simulink model "pid_control_aerobot"  (R2024a)
settings: Solver=ode1  StartTime=0.0  StopTime=inf  FixedStep=0.01  RelTol=1e-3
undefined symbols (not defined in the file or in its folder): DiscIntNeverNeededParam, pin_number, state
libraries: ros2lib x14, simulink x2, sharedtransform x1
settings Model: SimulationMode=external  Creator=dsai9  LastModifiedBy=dsai9
settings OptimizationCC: EnhancedBackFolding=on  PassReuseOutputArgsAs=Individual arguments  ZeroExternalMemoryAtStartup=off  ZeroInternalMemoryAtStartup=off  MaxStackSize=64  OptimizeBlockOrder=speed  DifferentSizesBufferReuse=on  OptimizationCustomize=off  EfficientTunableParamExpr=on
settings DebuggingCC: ParameterTunabilityLossMsg=error
settings HardwareCC: ProdBitPerLong=64  ProdLargestAtomicInteger=LongLong  ProdLargestAtomicFloat=Double  ProdLongLongMode=on  ProdHWDeviceType=ARM Compatible->ARM Cortex-A (64-bit)
settings SFSimCC: MATLABDynamicMemAlloc=off
settings RTWCC: Description=Embedded Coder  SystemTargetFile=ert.tlc  HardwareBoard=Robot Operating System 2 (ROS 2)  TLCOptions="-aInlineSetEventsForThisBaseRateFcn=TLC_FALSE -aSuppressMultiTaskScheduler=TLC_FALSE  -aRateBasedStepFcn=0"  TemplateMakefile=ert_default_tmf  Toolchain=Colcon Tools  TargetLang=C++  GPUComputeCapability=3.5
settings CodeAppCC: ForceParamTrailComments=on  IgnoreCustomStorageClasses=off  OperatorAnnotations=on  SimulinkDataObjDesc=on  SFDataObjDesc=on  InsertBlockDesc=on
settings ERTTargetCC: TargetLangStandard=C++11 (ISO)  ExtMode=on  ExtModeMexArgs='192.168.0.122' 0 17725  RootIOFormat=Structure reference

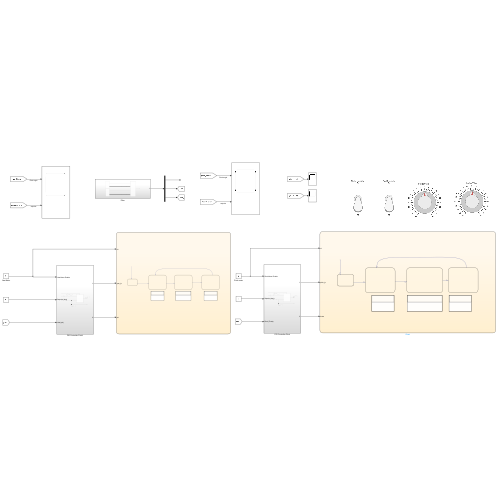
[thumbnail: Simulink's stored preview of the top-level diagram]
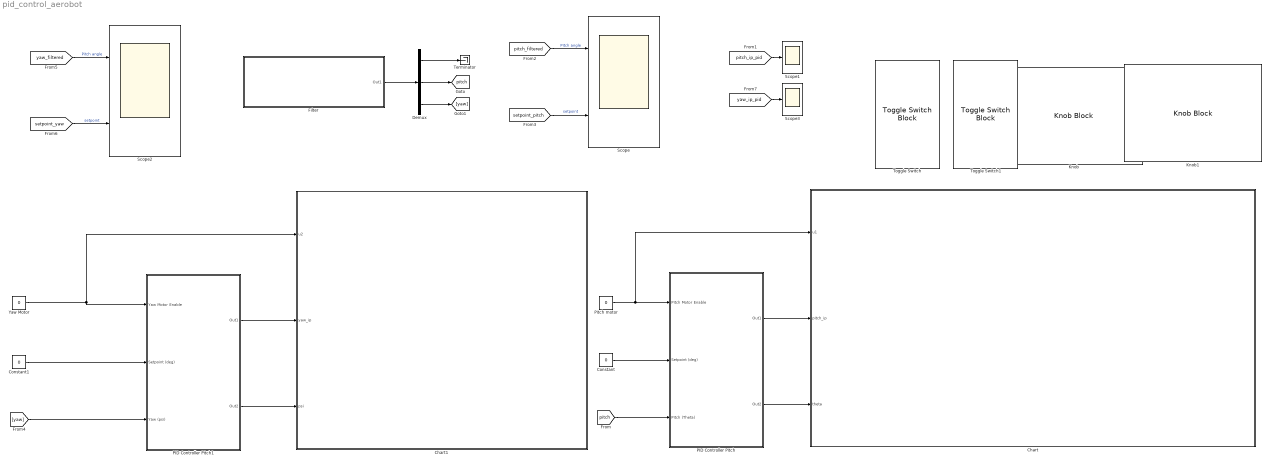
== system pid_control_aerobot ==
  Chart : Stateflow chart  TreatAsAtomicUnit=on
  Chart1 : Stateflow chart  TreatAsAtomicUnit=on
  Constant : Constant  Value=0
  Constant1 : Constant  Value=0
  Demux : Demux  Outputs=3
  Filter : Subsystem
  Knob : KnobBlock  ScaleMin=-40  ScaleMax=40
  Knob1 : KnobBlock  ScaleMin=-40  ScaleMax=40
  PID Controller Pitch : Subsystem
  PID Controller Pitch1 : Subsystem
  Pitch motor : Constant  Value=0  OutDataTypeStr=boolean
  Scope : Scope  NumInputPorts=2
  Scope1 : Scope
  Scope2 : Scope  NumInputPorts=2
  Scope3 : Scope
  Terminator : Terminator
  Toggle Switch : ToggleSwitchBlock
      settings: Values={{'Off', 'On'}, [0 1]}
  Toggle Switch1 : ToggleSwitchBlock
      settings: Values={{'Off', 'On'}, [0 1]}
  Yaw Motor : Constant  Value=0  OutDataTypeStr=boolean
  tag scope: pitch=global
  wires:
  [pitch_ip_pid] -> Scope1/1
  Filter/1(Out1) -> Demux/1
  Demux/3 -> [yaw]
  [pitch_filtered] -> Scope/1  "Pitch angle"
  Demux/1 -> Terminator/1
  Yaw Motor/1 -> Chart1/1(u2), PID Controller Pitch1/1(Yaw Motor Enable)
  [setpoint_pitch] -> Scope/2  "setpoint"
  Demux/2 -> [pitch]
  Pitch motor/1 -> Chart/1(u1), PID Controller Pitch/1(Pitch Motor Enable)
  PID Controller Pitch/2(Out2) -> Chart/3(theta)
  Constant/1 -> PID Controller Pitch/2(Setpoint (deg))
  [pitch] -> PID Controller Pitch/3(Pitch (Theta))
  PID Controller Pitch/1(Out1) -> Chart/2(pitch_ip)
  PID Controller Pitch1/1(Out1) -> Chart1/2(yaw_ip)
  PID Controller Pitch1/2(Out2) -> Chart1/3(psi)
  Constant1/1 -> PID Controller Pitch1/2(Setpoint (deg))
  [yaw] -> PID Controller Pitch1/3(Yaw (psi))
  [setpoint_yaw] -> Scope2/2  "setpoint"
  [yaw_filtered] -> Scope2/1  "Pitch angle"
  [yaw_ip_pid] -> Scope3/1

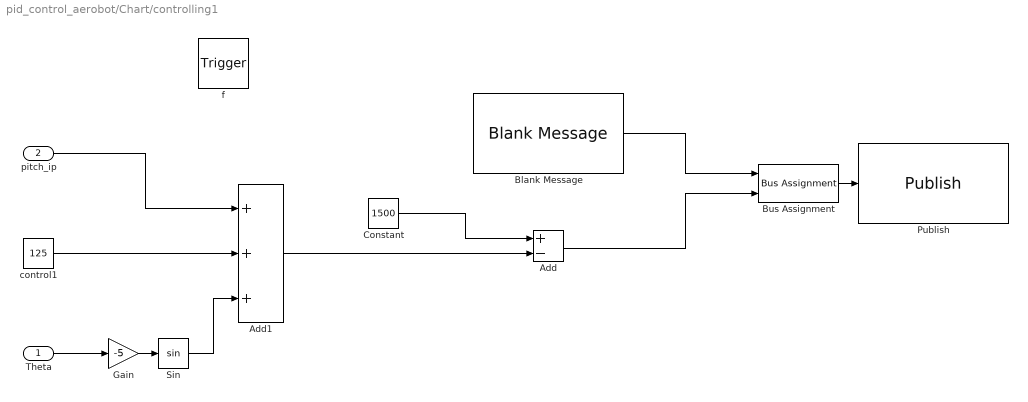
== system pid_control_aerobot/Chart/controlling1 ==
  Theta : Inport  OutDataTypeStr=double  PortDimensions=1
  pitch_ip : Inport  Port=2  OutDataTypeStr=double  PortDimensions=1  LockScale=on
  f : TriggerPort  TriggerType=function-call  VariantControl=(inherit)
      settings: CopyFcn=Stateflow.SLINSF.SimulinkMan.removeBlockPreDeleteFcn  PreDeleteFcn=Stateflow.SLINSF.SimulinkMan.unsafePredeleteFcn
  Add : Sum  Inputs=+-
  Add1 : Sum  Inputs=+++
  Blank Message : ros2lib/Blank Message  messageClass=Message  entityType=std_msgs/Float64  messageType=std_msgs/Float64  SampleTime=inf
  Bus Assignment : BusAssignment  AssignedSignals=data
  Constant : Constant  Value=1500
  Gain : Gain  Gain=-5
  Publish : ros2lib/Publish  topicSource=Select from ROS network  topic=/esc_command1  messageType=std_msgs/Float64  QOSHistory=Keep last  QOSDepth=10  QOSReliability=Reliable  QOSDurability=Volatile  QOSDeadline=Inf  QOSLifespan=Inf  QOSLiveliness=Automatic  QOSLeaseDuration=Inf  QOSAvoidROSNamespaceConventions=off
  Sin : Trigonometry
  control1 : Constant  Value=125
  wires:
  Constant/1 -> Add/1
  Bus Assignment/1 -> Publish/1
  Blank Message/1 -> Bus Assignment/1
  Add/1 -> Bus Assignment/2
  control1/1 -> Add1/2
  Add1/1 -> Add/2
  pitch_ip/1 -> Add1/1
  Gain/1 -> Sin/1
  Sin/1 -> Add1/3
  Theta/1 -> Gain/1

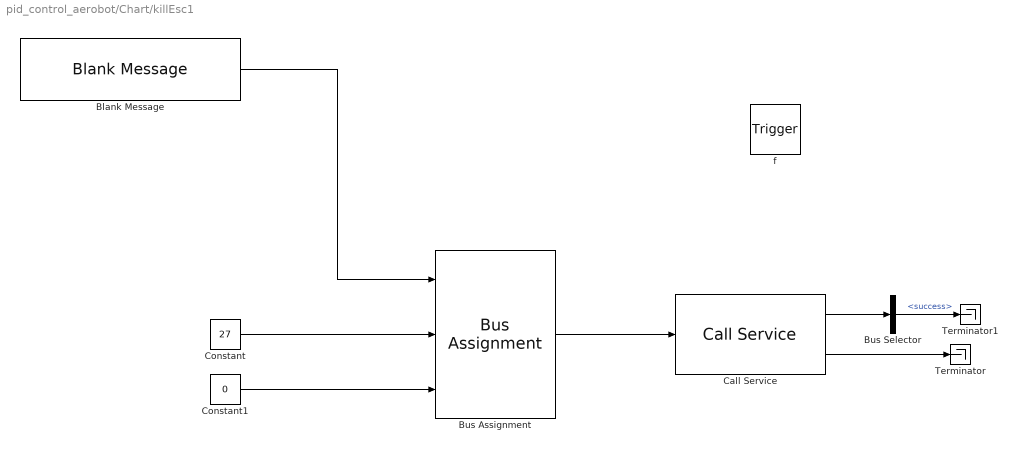
== system pid_control_aerobot/Chart/killEsc1 ==
  f : TriggerPort  TriggerType=function-call  VariantControl=(inherit)
      settings: CopyFcn=Stateflow.SLINSF.SimulinkMan.removeBlockPreDeleteFcn  PreDeleteFcn=Stateflow.SLINSF.SimulinkMan.unsafePredeleteFcn
  Blank Message : ros2lib/Blank Message  messageClass=Service Request  entityType=aerobot_interfaces/EscSrv  messageType=aerobot_interfaces/EscSrvRequest  SampleTime=inf
  Bus Assignment : BusAssignment  AssignedSignals=pin_number,state
  Bus Selector : BusSelector  OutputSignals=success
  Call Service : ros2lib/Call Service  topicSource=Select from ROS network  service=/arm_pitch  serviceType=aerobot_interfaces/EscSrv  connectionTimeout=5  ShowErrorCodeOutput=on  legacyBusStruct=off  QOSHistory=Keep last  QOSDepth=1  QOSReliability=Reliable  QOSDurability=Volatile  QOSDeadline=Inf  QOSLifespan=Inf  QOSLiveliness=Automatic  QOSLeaseDuration=Inf  QOSAvoidROSNamespaceConventions=off
  Constant : Constant  Value=27  OutDataTypeStr=int8
  Constant1 : Constant  Value=0  OutDataTypeStr=boolean
  Terminator : Terminator
  Terminator1 : Terminator
  wires:
  Bus Assignment/1 -> Call Service/1
  Blank Message/1 -> Bus Assignment/1
  Call Service/1 -> Bus Selector/1
  Bus Selector/1 -> Terminator1/1  "<success>"
  Call Service/2 -> Terminator/1
  Constant/1 -> Bus Assignment/2
  Constant1/1 -> Bus Assignment/3

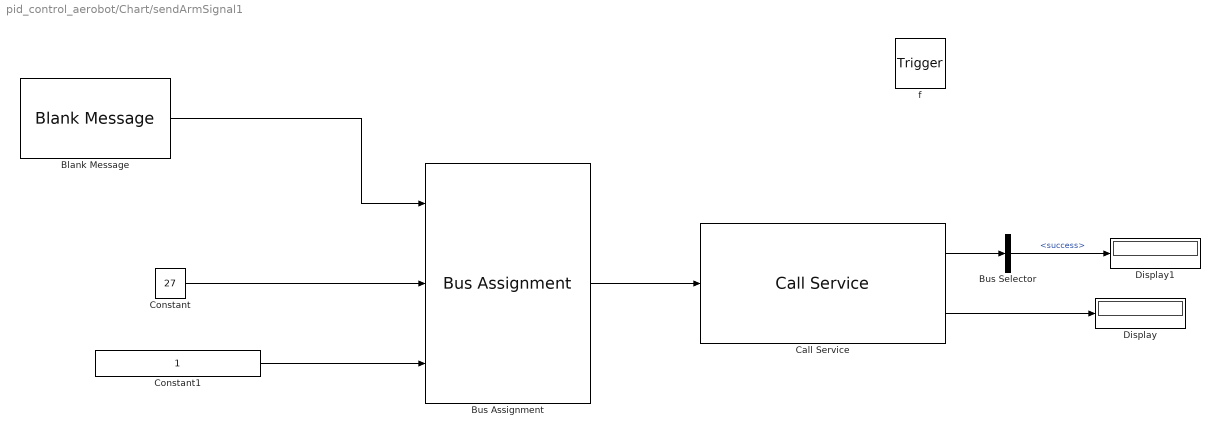
== system pid_control_aerobot/Chart/sendArmSignal1 ==
  f : TriggerPort  TriggerType=function-call  VariantControl=(inherit)
      settings: CopyFcn=Stateflow.SLINSF.SimulinkMan.removeBlockPreDeleteFcn  PreDeleteFcn=Stateflow.SLINSF.SimulinkMan.unsafePredeleteFcn
  Blank Message : ros2lib/Blank Message  messageClass=Service Request  entityType=aerobot_interfaces/EscSrv  messageType=aerobot_interfaces/EscSrvRequest  SampleTime=inf
  Bus Assignment : BusAssignment  AssignedSignals=pin_number,state
  Bus Selector : BusSelector  OutputSignals=success
  Call Service : ros2lib/Call Service  topicSource=Select from ROS network  service=/arm_pitch  serviceType=aerobot_interfaces/EscSrv  connectionTimeout=5  ShowErrorCodeOutput=on  legacyBusStruct=off  QOSHistory=Keep last  QOSDepth=1  QOSReliability=Reliable  QOSDurability=Volatile  QOSDeadline=Inf  QOSLifespan=Inf  QOSLiveliness=Automatic  QOSLeaseDuration=Inf  QOSAvoidROSNamespaceConventions=off
  Constant : Constant  Value=27  OutDataTypeStr=int8
  Constant1 : Constant  OutDataTypeStr=boolean
  Display : Display
  Display1 : Display
  wires:
  Bus Assignment/1 -> Call Service/1
  Blank Message/1 -> Bus Assignment/1
  Constant/1 -> Bus Assignment/2
  Constant1/1 -> Bus Assignment/3
  Call Service/1 -> Bus Selector/1
  Bus Selector/1 -> Display1/1  "<success>"
  Call Service/2 -> Display/1

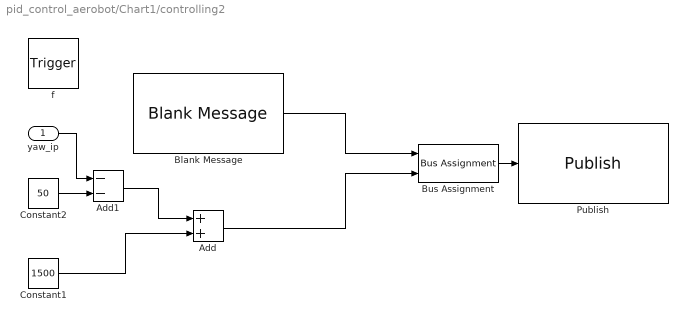
== system pid_control_aerobot/Chart1/controlling2 ==
  yaw_ip : Inport  OutDataTypeStr=double  PortDimensions=1
  f : TriggerPort  TriggerType=function-call  VariantControl=(inherit)
      settings: CopyFcn=Stateflow.SLINSF.SimulinkMan.removeBlockPreDeleteFcn  PreDeleteFcn=Stateflow.SLINSF.SimulinkMan.unsafePredeleteFcn
  Add : Sum
  Add1 : Sum  Inputs=--
  Blank Message : ros2lib/Blank Message  messageClass=Message  entityType=std_msgs/Float64  messageType=std_msgs/Float64  SampleTime=inf
  Bus Assignment : BusAssignment  AssignedSignals=data
  Constant1 : Constant  Value=1500
  Constant2 : Constant  Value=50
  Publish : ros2lib/Publish  topicSource=Select from ROS network  topic=/esc_command2  messageType=std_msgs/Float64  QOSHistory=Keep last  QOSDepth=10  QOSReliability=Reliable  QOSDurability=Volatile  QOSDeadline=Inf  QOSLifespan=Inf  QOSLiveliness=Automatic  QOSLeaseDuration=Inf  QOSAvoidROSNamespaceConventions=off
  wires:
  Bus Assignment/1 -> Publish/1
  Blank Message/1 -> Bus Assignment/1
  Add/1 -> Bus Assignment/2
  Constant1/1 -> Add/2
  Constant2/1 -> Add1/2
  Add1/1 -> Add/1
  yaw_ip/1 -> Add1/1

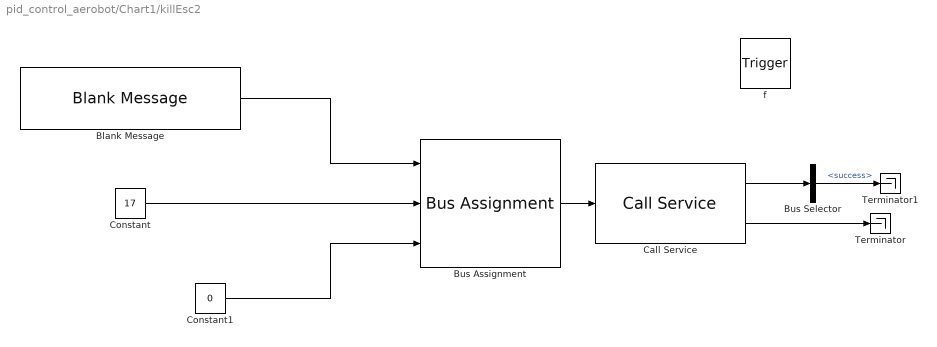
== system pid_control_aerobot/Chart1/killEsc2 ==
  f : TriggerPort  TriggerType=function-call  VariantControl=(inherit)
      settings: CopyFcn=Stateflow.SLINSF.SimulinkMan.removeBlockPreDeleteFcn  PreDeleteFcn=Stateflow.SLINSF.SimulinkMan.unsafePredeleteFcn
  Blank Message : ros2lib/Blank Message  messageClass=Service Request  entityType=aerobot_interfaces/EscSrv  messageType=aerobot_interfaces/EscSrvRequest  SampleTime=inf
  Bus Assignment : BusAssignment  AssignedSignals=pin_number,state
  Bus Selector : BusSelector  OutputSignals=success
  Call Service : ros2lib/Call Service  topicSource=Select from ROS network  service=/arm_yaw  serviceType=aerobot_interfaces/EscSrv  connectionTimeout=5  ShowErrorCodeOutput=on  legacyBusStruct=off  QOSHistory=Keep last  QOSDepth=1  QOSReliability=Reliable  QOSDurability=Volatile  QOSDeadline=Inf  QOSLifespan=Inf  QOSLiveliness=Automatic  QOSLeaseDuration=Inf  QOSAvoidROSNamespaceConventions=off
  Constant : Constant  Value=17  OutDataTypeStr=int8
  Constant1 : Constant  Value=0  OutDataTypeStr=boolean
  Terminator : Terminator
  Terminator1 : Terminator
  wires:
  Bus Assignment/1 -> Call Service/1
  Blank Message/1 -> Bus Assignment/1
  Call Service/1 -> Bus Selector/1
  Bus Selector/1 -> Terminator1/1  "<success>"
  Call Service/2 -> Terminator/1
  Constant/1 -> Bus Assignment/2
  Constant1/1 -> Bus Assignment/3

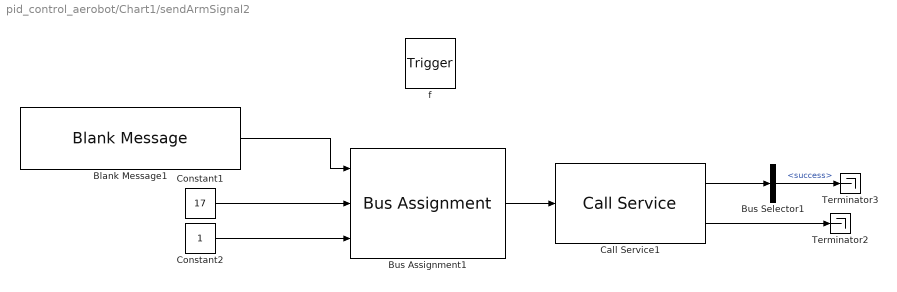
== system pid_control_aerobot/Chart1/sendArmSignal2 ==
  f : TriggerPort  TriggerType=function-call  VariantControl=(inherit)
      settings: CopyFcn=Stateflow.SLINSF.SimulinkMan.removeBlockPreDeleteFcn  PreDeleteFcn=Stateflow.SLINSF.SimulinkMan.unsafePredeleteFcn
  Blank Message1 : ros2lib/Blank Message  messageClass=Service Request  entityType=aerobot_interfaces/EscSrv  messageType=aerobot_interfaces/EscSrvRequest  SampleTime=inf
  Bus Assignment1 : BusAssignment  AssignedSignals=pin_number,state
  Bus Selector1 : BusSelector  OutputSignals=success
  Call Service1 : ros2lib/Call Service  topicSource=Select from ROS network  service=/arm_yaw  serviceType=aerobot_interfaces/EscSrv  connectionTimeout=5  ShowErrorCodeOutput=on  legacyBusStruct=off  QOSHistory=Keep last  QOSDepth=1  QOSReliability=Reliable  QOSDurability=Volatile  QOSDeadline=Inf  QOSLifespan=Inf  QOSLiveliness=Automatic  QOSLeaseDuration=Inf  QOSAvoidROSNamespaceConventions=off
  Constant1 : Constant  Value=17  OutDataTypeStr=int8
  Constant2 : Constant  OutDataTypeStr=boolean
  Terminator2 : Terminator
  Terminator3 : Terminator
  wires:
  Call Service1/1 -> Bus Selector1/1
  Bus Selector1/1 -> Terminator3/1  "<success>"
  Call Service1/2 -> Terminator2/1
  Constant1/1 -> Bus Assignment1/2
  Bus Assignment1/1 -> Call Service1/1
  Blank Message1/1 -> Bus Assignment1/1
  Constant2/1 -> Bus Assignment1/3

== system pid_control_aerobot/Filter ==
  Subscribe : ros2lib/Subscribe  topicSource=Select from ROS network  topic=/imu/data  messageType=sensor_msgs/Imu  sampleTime=0.01  QOSHistory=Keep last  QOSDepth=10  QOSReliability=Reliable  QOSDurability=Volatile  QOSDeadline=Inf  QOSLifespan=Inf  QOSLiveliness=Automatic  QOSLeaseDuration=Inf  QOSAvoidROSNamespaceConventions=off
  Subscribe1 : ros2lib/Subscribe  topicSource=Select from ROS network  topic=/mag/data  messageType=sensor_msgs/MagneticField  sampleTime=0.01  QOSHistory=Keep last  QOSDepth=10  QOSReliability=Reliable  QOSDurability=Volatile  QOSDeadline=Inf  QOSLifespan=Inf  QOSLiveliness=Automatic  QOSLeaseDuration=Inf  QOSAvoidROSNamespaceConventions=off
  Subsystem : Subsystem  mask{alpha=0}
  Out1 : Outport
  wires:
  Subscribe1/2 -> Subsystem/4(In4)
  Subscribe/2 -> Subsystem/2(In2)
  Subscribe/1 -> Subsystem/1(In1)
  Subscribe1/1 -> Subsystem/3(In3)
  Subsystem/1(Out1) -> Out1/1

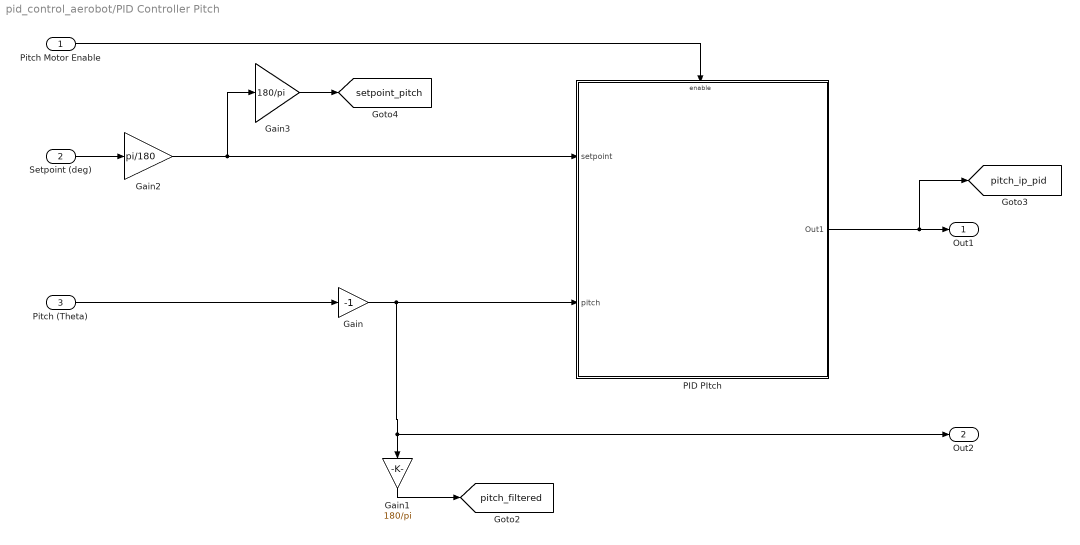
== system pid_control_aerobot/PID Controller Pitch ==
  Pitch Motor Enable : Inport
  Setpoint (deg) : Inport  Port=2
  Pitch (Theta) : Inport  Port=3
  Gain : Gain  Gain=-1
  Gain1 : Gain  Gain=180/pi
  Gain2 : Gain  Gain=pi/180
  Gain3 : Gain  Gain=180/pi
  PID PItch : Subsystem
  Out1 : Outport
  Out2 : Outport  Port=2
  tag scope: pitch_filtered=global, pitch_ip_pid=global, setpoint_pitch=global
  wires:
  Pitch (Theta)/1 -> Gain/1
  Gain/1 -> PID PItch/2(pitch), Out2/1, Gain1/1
  Gain1/1 -> [pitch_filtered]
  PID PItch/1(Out1) -> Out1/1, [pitch_ip_pid]
  Pitch Motor Enable/1 -> PID PItch/Enable
  Gain2/1 -> PID PItch/1(setpoint), Gain3/1
  Gain3/1 -> [setpoint_pitch]
  Setpoint (deg)/1 -> Gain2/1

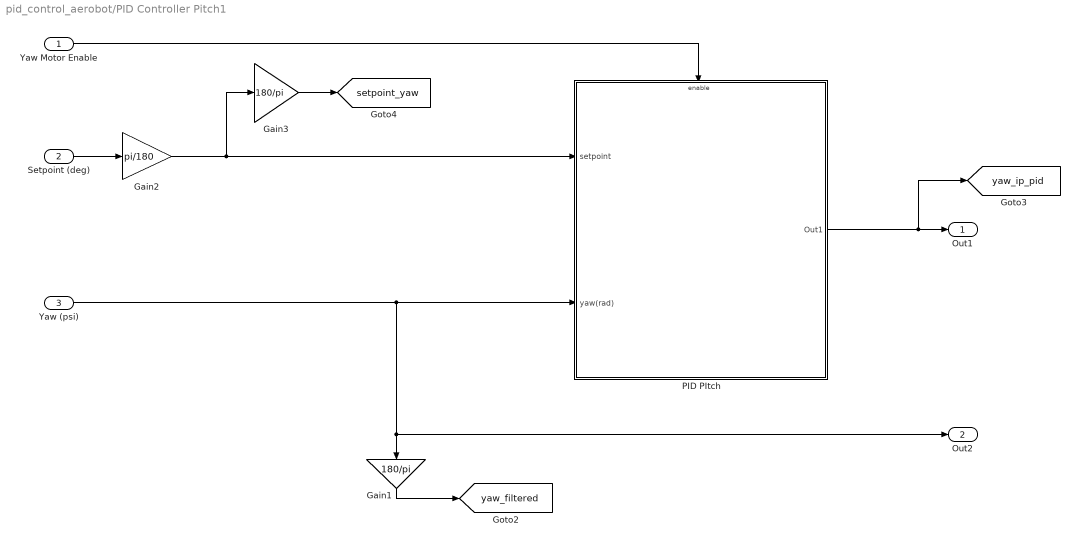
== system pid_control_aerobot/PID Controller Pitch1 ==
  Yaw Motor Enable : Inport
  Setpoint (deg) : Inport  Port=2
  Yaw (psi) : Inport  Port=3
  Gain1 : Gain  Gain=180/pi
  Gain2 : Gain  Gain=pi/180
  Gain3 : Gain  Gain=180/pi
  PID PItch : Subsystem
  Out1 : Outport
  Out2 : Outport  Port=2
  tag scope: setpoint_yaw=global, yaw_filtered=global, yaw_ip_pid=global
  wires:
  Setpoint (deg)/1 -> Gain2/1
  Gain3/1 -> [setpoint_yaw]
  Gain2/1 -> Gain3/1, PID PItch/1(setpoint)
  Yaw Motor Enable/1 -> PID PItch/Enable
  PID PItch/1(Out1) -> [yaw_ip_pid], Out1/1
  Gain1/1 -> [yaw_filtered]
  Yaw (psi)/1 -> PID PItch/2(yaw(rad)), Out2/1, Gain1/1

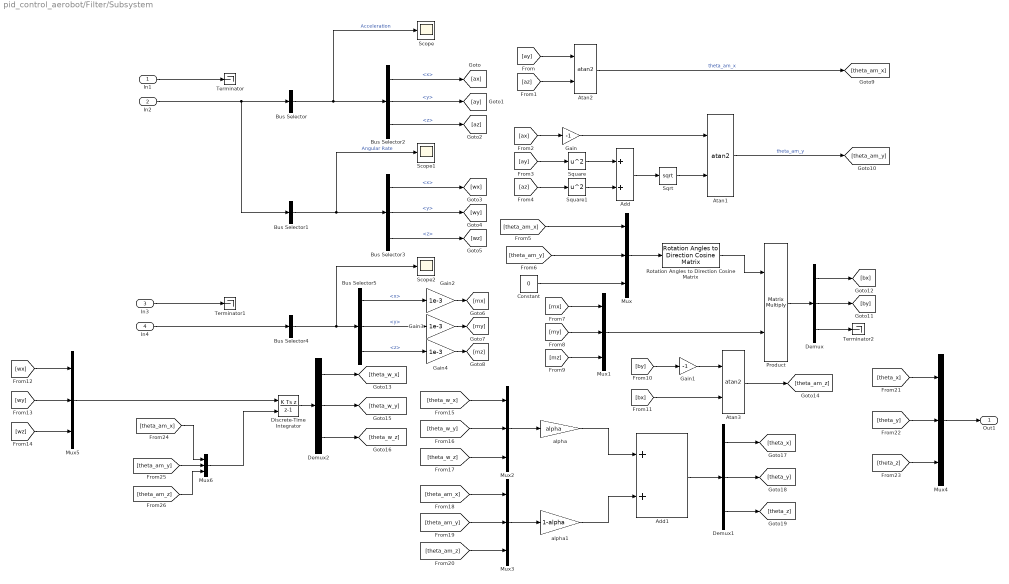
== system pid_control_aerobot/Filter/Subsystem ==
  In1 : Inport
  In2 : Inport  Port=2
  In3 : Inport  Port=3
  In4 : Inport  Port=4
  Add : Sum
  Add1 : Sum
  Atan1 : Trigonometry  Operator=atan2
  Atan2 : Trigonometry  Operator=atan2
  Atan3 : Trigonometry  Operator=atan2
  Bus Selector : BusSelector  OutputSignals=linear_acceleration.x,linear_acceleration.y,linear_acceleration.z  OutputAsBus=on
  Bus Selector1 : BusSelector  OutputSignals=angular_velocity.x,angular_velocity.y,angular_velocity.z  OutputAsBus=on
  Bus Selector2 : BusSelector  OutputSignals=x,y,z
  Bus Selector3 : BusSelector  OutputSignals=x,y,z
  Bus Selector4 : BusSelector  OutputSignals=magnetic_field.x,magnetic_field.y,magnetic_field.z  OutputAsBus=on
  Bus Selector5 : BusSelector  OutputSignals=x,y,z
  Constant : Constant  Value=0
  Demux : Demux  Outputs=3
  Demux1 : Demux  Outputs=3
  Demux2 : Demux  Outputs=3
  Discrete-Time Integrator : DiscreteIntegrator  IntegratorMethod=Integration: Backward Euler  gainval=3  InitialConditionSource=external  InitialCondition=zeros(3,1)  SampleTime=-1  ICPrevOutput=DiscIntNeverNeededParam  ICPrevScaledInput=DiscIntNeverNeededParam
  Gain : Gain  Gain=-1
  Gain1 : Gain  Gain=-1
  Gain2 : Gain  Gain=1e-3
  Gain3 : Gain  Gain=1e-3
  Gain4 : Gain  Gain=1e-3
  Mux{,1..6} (7 alike) : Mux  Inputs=3
  Product : Product  Multiplication=Matrix(*)
  Rotation Angles to Direction Cosine Matrix : sharedtransform/Rotation Angles to Direction Cosine Matrix  rotationOrder=YXZ  aMode=aMode
  Scope : Scope
  Scope1 : Scope
  Scope2 : Scope
  Sqrt : Sqrt
  Square : Math  Operator=square
  Square1 : Math  Operator=square
  Terminator : Terminator
  Terminator1 : Terminator
  Terminator2 : Terminator
  alpha : Gain  Gain=alpha
  alpha1 : Gain  Gain=1-alpha
  Out1 : Outport
  wires:
  Mux1/1 -> Product/2
  Product/1 -> Demux/1
  Rotation Angles to Direction Cosine Matrix/1 -> Product/1
  Bus Selector2/2 -> [ay]  "<y>"
  [wx] -> Mux5/1
  [by] -> Gain1/1
  Demux/3 -> Terminator2/1
  Square1/1 -> Add/2
  Demux2/3 -> [theta_w_z]
  Bus Selector1/1 -> Scope1/1, Bus Selector3/1  "Angular Rate"
  Square/1 -> Add/1
  Bus Selector/1 -> Scope/1, Bus Selector2/1  "Acceleration"
  [theta_y] -> Mux4/2
  alpha/1 -> Add1/1
  [mx] -> Mux1/1
  [theta_am_x] -> Mux3/1
  Demux1/3 -> [theta_z]
  Gain/1 -> Atan1/1
  Constant/1 -> Mux/3
  Demux/1 -> [bx]
  Bus Selector5/3 -> Gain4/1  "<z>"
  Bus Selector5/1 -> Gain2/1  "<x>"
  In2/1 -> Bus Selector1/1, Bus Selector/1
  Add/1 -> Sqrt/1
  [az] -> Atan2/2
  [theta_am_y] -> Mux/2
  [my] -> Mux1/2
  [ax] -> Gain/1
  Gain1/1 -> Atan3/1
  [ay] -> Atan2/1
  Bus Selector3/2 -> [wy]  "<y>"
  Bus Selector3/3 -> [wz]  "<z>"
  Demux2/2 -> [theta_w_y]
  Atan2/1 -> [theta_am_x]  "theta_am_x"
  Demux1/2 -> [theta_y]
  Mux3/1 -> alpha1/1
  Bus Selector2/3 -> [az]  "<z>"
  Bus Selector5/2 -> Gain3/1  "<y>"
  [theta_w_z] -> Mux2/3
  Bus Selector2/1 -> [ax]  "<x>"
  [az] -> Square1/1
  Atan1/1 -> [theta_am_y]  "theta_am_y"
  Bus Selector3/1 -> [wx]  "<x>"
  [theta_am_y] -> Mux3/2
  Sqrt/1 -> Atan1/2
  [ay] -> Square/1
  Mux/1 -> Rotation Angles to Direction Cosine Matrix/1
  Mux4/1 -> Out1/1
  [mz] -> Mux1/3
  [theta_am_x] -> Mux/1
  Atan3/1 -> [theta_am_z]
  Demux1/1 -> [theta_x]
  [theta_am_z] -> Mux3/3
  [theta_z] -> Mux4/3
  [theta_x] -> Mux4/1
  Demux2/1 -> [theta_w_x]
  Add1/1 -> Demux1/1
  Mux2/1 -> alpha/1
  [theta_w_x] -> Mux2/1
  [wz] -> Mux5/3
  [theta_w_y] -> Mux2/2
  [bx] -> Atan3/2
  alpha1/1 -> Add1/2
  Demux/2 -> [by]
  [wy] -> Mux5/2
  In4/1 -> Bus Selector4/1
  In1/1 -> Terminator/1
  In3/1 -> Terminator1/1
  Bus Selector4/1 -> Scope2/1, Bus Selector5/1
  Mux5/1 -> Discrete-Time Integrator/1
  Discrete-Time Integrator/1 -> Demux2/1
  Gain2/1 -> [mx]
  Gain3/1 -> [my]
  Gain4/1 -> [mz]
  [theta_am_x] -> Mux6/1
  [theta_am_y] -> Mux6/2
  [theta_am_z] -> Mux6/3
  Mux6/1 -> Discrete-Time Integrator/2

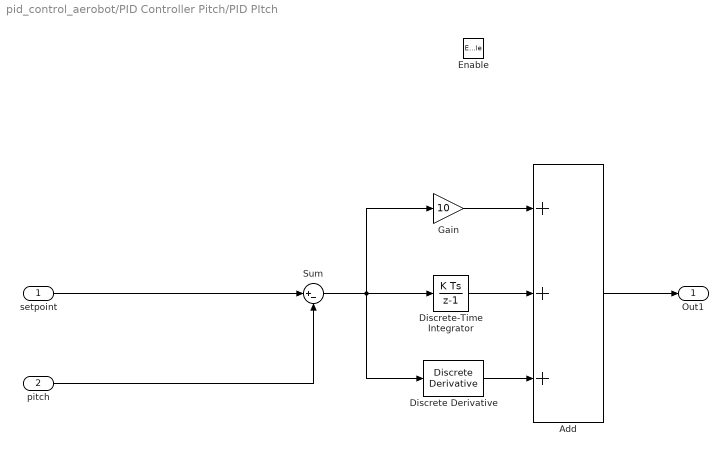
== system pid_control_aerobot/PID Controller Pitch/PID PItch ==
  setpoint : Inport
  pitch : Inport  Port=2
  Enable : EnablePort
  Add : Sum  Inputs=+++
  Discrete Derivative : simulink/Discrete/Discrete Derivative  gainval=1  ICPrevScaledInput=0.0  OutMin=[]  OutMax=[]  OutDataType=fixdt(1, 16)  OutScaling=2^-10  DoSatur=off
  Discrete-Time Integrator : DiscreteIntegrator  gainval=1.5  SampleTime=-1  ICPrevOutput=DiscIntNeverNeededParam  ICPrevScaledInput=DiscIntNeverNeededParam
  Gain : Gain  Gain=10
  Sum : Sum  Inputs=|+-
  Out1 : Outport
  wires:
  setpoint/1 -> Sum/1
  Discrete-Time Integrator/1 -> Add/2
  Gain/1 -> Add/1
  Sum/1 -> Discrete Derivative/1, Discrete-Time Integrator/1, Gain/1
  Add/1 -> Out1/1
  Discrete Derivative/1 -> Add/3
  pitch/1 -> Sum/2

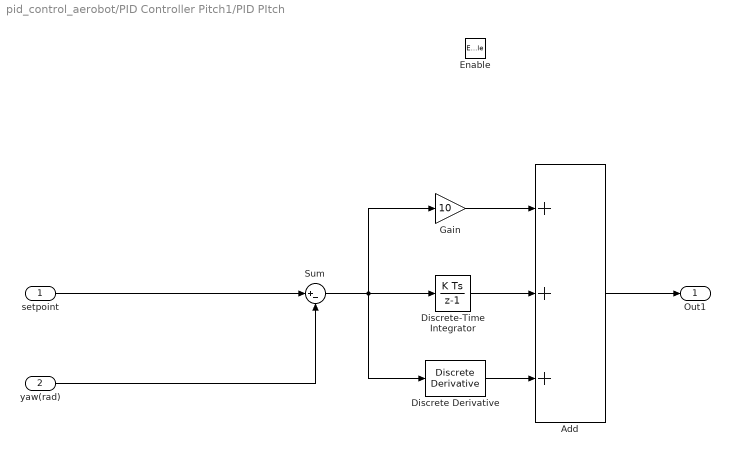
== system pid_control_aerobot/PID Controller Pitch1/PID PItch ==
  setpoint : Inport
  yaw(rad) : Inport  Port=2
  Enable : EnablePort
  Add : Sum  Inputs=+++
  Discrete Derivative : simulink/Discrete/Discrete Derivative  gainval=5  ICPrevScaledInput=0.0  OutMin=[]  OutMax=[]  OutDataType=fixdt(1, 16)  OutScaling=2^-10  DoSatur=off
  Discrete-Time Integrator : DiscreteIntegrator  gainval=1.5  SampleTime=-1  ICPrevOutput=DiscIntNeverNeededParam  ICPrevScaledInput=DiscIntNeverNeededParam
  Gain : Gain  Gain=10
  Sum : Sum  Inputs=|+-
  Out1 : Outport
  wires:
  yaw(rad)/1 -> Sum/2
  Discrete Derivative/1 -> Add/3
  Add/1 -> Out1/1
  Sum/1 -> Gain/1, Discrete-Time Integrator/1, Discrete Derivative/1
  Gain/1 -> Add/1
  Discrete-Time Integrator/1 -> Add/2
  setpoint/1 -> Sum/1

== stateflow chart pid_control_aerobot/Chart1 ==
  state ARM1
    entry:
    disp('ARMING ESC..')
    during:
    sendArmSignal2();
    y2 = 1;
  state Command1
    entry:
    disp('Send Commands')
    during:
    controlling2(yaw_ip);
  state Kill1
    entry:
    killEsc2();
  state Init1
    entry, during:
    k2 = u2;
  state sendArmSignal2 [function]
  state controlling2(yaw_ip) [function]
  state killEsc2 [function]
  (default) -> Init1
  Kill1 -> ARM1 : [u2 == 1]
  Command1 -> Kill1 : [u2==0]
  ARM1 -> Command1 : [y2 == 1]
  Init1 -> ARM1 : [k2 == 1]
  data: yaw_ip function_input double size=1; u2 input; k2 local; y2 local; yaw_ip input; psi input

== stateflow chart pid_control_aerobot/Chart ==
  state ARM
    entry:
    disp('ARMING ESC..')
    during:
    sendArmSignal1();
    y1 = 1;
  state Command
    entry:
    disp('Send Commands')
    during:
    controlling1(theta, pitch_ip);
  state Kill
    entry:
    killEsc1();
  state Init
    entry, during:
    k1 = u1;
  state sendArmSignal1 [function]
  state controlling1(Theta,pitch_ip) [function]
  state killEsc1 [function]
  Kill -> ARM : [u1 == 1]
  (default) -> Init
  Command -> Kill : [u1==0]
  ARM -> Command : [y1 == 1]
  Init -> ARM : [k1 == 1]
  data: Theta function_input double size=1; pitch_ip function_input double size=1; k1 local; y1 local int8 size=1 =0; u1 input; pitch_ip input; theta input double size=1
